simulink model "example"  (R2022b)
settings: Solver=VariableStepAuto  StartTime=0.0  StopTime=10.0  RelTol=1e-3
settings Model: Creator=Utente  LastModifiedBy=Utente
settings SFSimCC: SimCustomHeaderCode="#include \"header.h\""  SimUserSources=souce.c  CustomCodeGlobalsAsFunctionIO=on

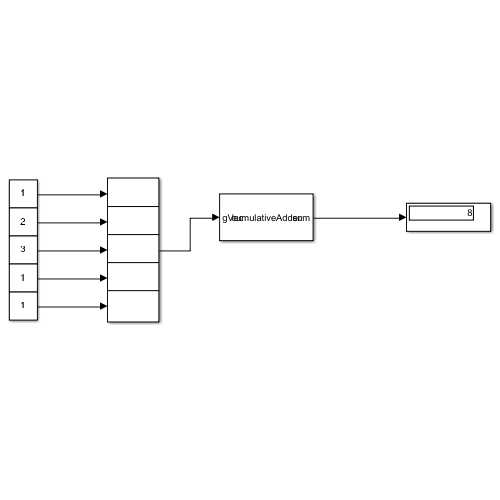
[thumbnail: Simulink's stored preview of the top-level diagram]
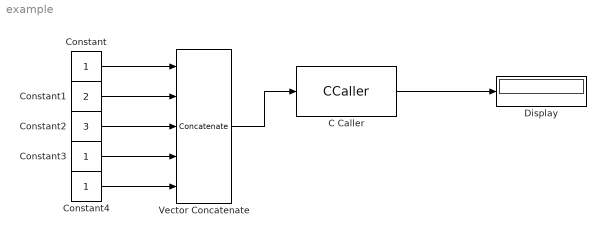
== system example ==
  C Caller : CCaller  FunctionName=cumulativeAdder  PortSpecificationStruct="%)30     .    N ,   8    (     @         %    \"     (    !     0         %  0 \"0    $    _    07)G3F%M90  4&]R=$YA;64 4V-O<&4     26YD97@     5'EP90      4VEZ90      27-';&]B86P   X    P    !@    @    $          4    (     0    0    !         !  ! !G5F5C#@   #     &    \"     0         !0    @    !    !     $         $  $ &=696,.    .     8    (    !          %    \"     $    %     0         0    !0   $EN<'5T    #@   #@    &    \"     8         !0    @    !     0    $         \"0    @               X    X    !@    @    $          4    (     0    8    !         !     &    9&]U8FQE   .    ,     8    (    !          %    \"     $    !     0         0  $ -0    X    P    !@    @    ) @        4    (     0    $    !          (  0 !    #@   #     &    \"     0         !0    @    !     P    $         $  # '-U;0 .    ,     8    (    !          %    \"     $    #     0         0  , <W5M  X    X    !@    @    $          4    (     0    8    !         !     &    3W5T<'5T   .    .     8    (    !@         %    \"     $    !     0         )    \"               #@   #@    &    \"     0         !0    @    !    !@    $         $     8   !D;W5B;&4   X    P    !@    @    $          4    (     0    $    !         !   0 Q    #@   #     &    \"     D\"        !0    @    !     0    $          @ !  $"
  Constant : Constant
  Constant1 : Constant  Value=2
  Constant2 : Constant  Value=3
  Constant3 : Constant
  Constant4 : Constant
  Display : Display
  Vector Concatenate : Concatenate  NumInputs=5
  wires:
  C Caller/1 -> Display/1
  Vector Concatenate/1 -> C Caller/1
  Constant/1 -> Vector Concatenate/1
  Constant1/1 -> Vector Concatenate/2
  Constant2/1 -> Vector Concatenate/3
  Constant3/1 -> Vector Concatenate/4
  Constant4/1 -> Vector Concatenate/5
